simulink model "l21"  (R2023a)
settings: Solver=VariableStepAuto  StartTime=0.0  StopTime=10.0  RelTol=1e-3
settings Model: Creator=Admin  LastModifiedBy=ввв
settings DebuggingCC: UnconnectedInputMsg=warning  UnconnectedOutputMsg=warning  UnconnectedLineMsg=warning
settings ModelReferenceCC: EnableRefExpFcnMdlSchedulingChecks=on
settings RTWCC: DLArmComputeVersion=19.05

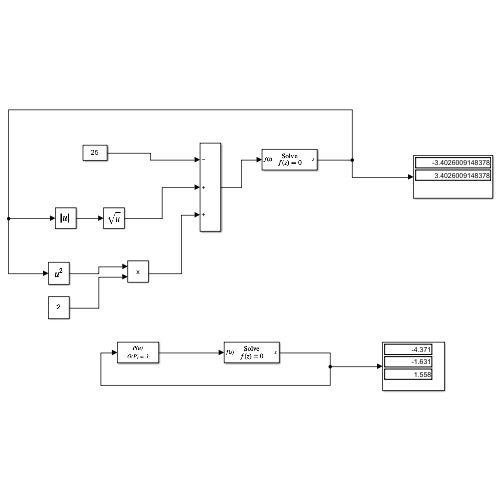
[thumbnail: Simulink's stored preview of the top-level diagram]
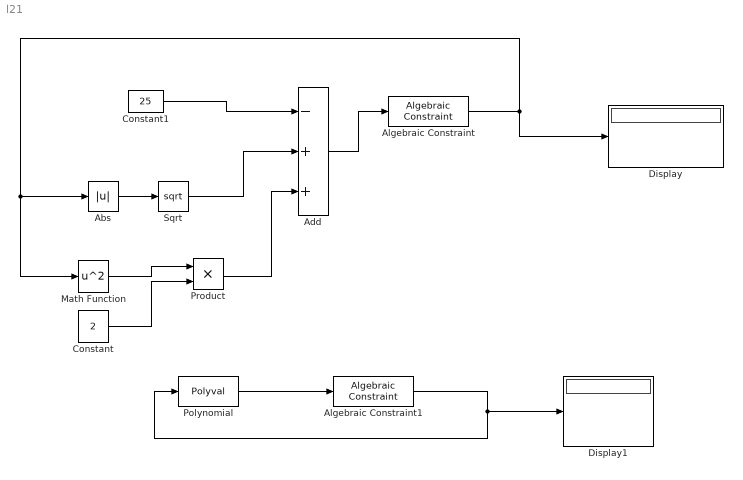
== system l21 ==
  Abs : Abs  SaturateOnIntegerOverflow=off
  Add : Sum  Inputs=-++
  Algebraic Constraint : AlgebraicConstraint  InitialGuess=[-3.4 3.4]
  Algebraic Constraint1 : AlgebraicConstraint  InitialGuess=[-4.4 -1.6 1.6]
  Constant : Constant  Value=2
  Constant1 : Constant  Value=25
  Display : Display
  Display1 : Display
  Math Function : Math  Operator=square
  Polynomial : Polyval  Coefs=[-0.9 -4 2 10]
  Product : Product
  Sqrt : Sqrt
  wires:
  Constant/1 -> Product/2
  Constant1/1 -> Add/1
  Sqrt/1 -> Add/2
  Product/1 -> Add/3
  Math Function/1 -> Product/1
  Algebraic Constraint/1 -> Abs/1, Math Function/1, Display/1
  Add/1 -> Algebraic Constraint/1
  Polynomial/1 -> Algebraic Constraint1/1
  Algebraic Constraint1/1 -> Polynomial/1, Display1/1
  Abs/1 -> Sqrt/1
